simulink subsystem "Full_Generator"  (R2020a)
settings: Solver=VariableStepAuto  StartTime=0.0  StopTime=10.0  RelTol=1e-3
undefined symbols (not defined in the file): radps2rpm, torque_pu2Nm, WT_Params
libraries: powerlib x8, Generator_Lib x3, fl_lib x2, Full_Generator_Lib x1, nesl_utility x1
settings Model: Creator=Luke  LastModifiedBy=Luke

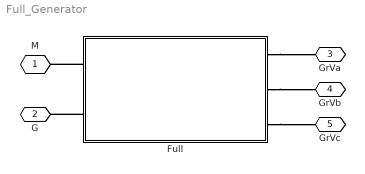
== system Full_Generator ==
  Full : Subsystem
  M : PMIOPort  Tag=PMCPort  Side=Left
  G : PMIOPort  Port=2  Side=Left
  GrVa : PMIOPort  Port=3  Side=Right
  GrVb : PMIOPort  Port=4  Side=Right
  GrVc : PMIOPort  Port=5  Side=Right
  connections:
  Full/RConn1 -- GrVa/RConn1
  Full/RConn2 -- GrVb/RConn1
  Full/RConn3 -- GrVc/RConn1
  Full/LConn1 -- M/RConn1
  Full/LConn2 -- G/RConn1

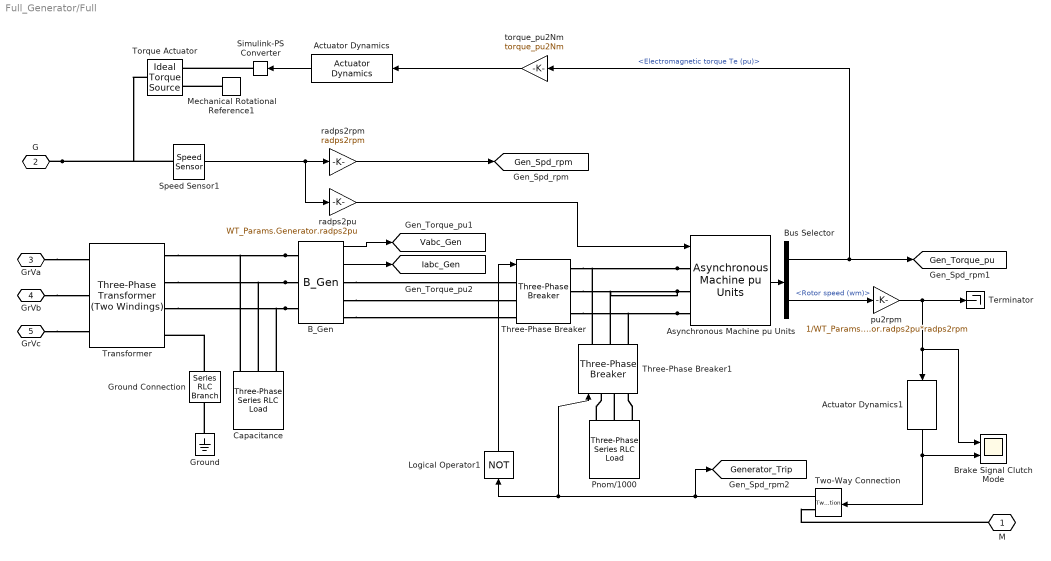
== system Full_Generator/Full ==
  Actuator Dynamics : Generator_Lib/Simple/Actuator Dynamics  b=WT_Params.Generator.generator_time_constant  x_initial=0
  Actuator Dynamics1 : Generator_Lib/Simple/Actuator Dynamics  b=WT_Params.Generator.generator_time_constant  x_initial=0
  Asynchronous Machine pu Units : powerlib/Machines/Asynchronous Machine pu Units  RotorType=Squirrel-cage  PresetModel=No  MechanicalLoad=Speed w  ShowDetailedParameters=on  ReferenceFrame=Rotor  Units=pu  MeasurementBus=off  NominalParameters=|  Stator=|  Rotor=|  Cage1=[0.01909 0.0397]  Cage2=[0.01909 0.0397]  Lm=WT_Params.Generator.mutual_inductance  Mechanical=[0.09526 0.05479 2]  PolePairs=2  InitialConditions=[1 0 0 0 0 0 0 0]  SimulateSaturation=off  Saturation="[0.212,0.4201,0.8125,1.0979,1.4799,2.2457,3.2586,4.5763,6.4763 ;   0.5,0.7,0.9,1,1.1,1.2 ,1.3,1.4,1.5]"  LoadFlowParameters=0  TsPowergui=0  TsBlock=-1  IterativeModel=Trapezoidal non iterative  IterativeDiscreteModel=Trapezoidal non iterative  Pmec=0
      NominalParameters=|
      | [WT_Params.Generator.nominal_power WT_Params.Generator.voltage
      | WT_Params.Generator.frequency]
      Stator=|
      | [WT_Params.Generator.Stator.resistance
      | WT_Params.Generator.Stator.inductance]
      Rotor=|
      | [WT_Params.Generator.Rotor.resistance
      | WT_Params.Generator.Rotor.inductance]
      settings: SourceProductBaseCode=PS
  B_Gen : Full_Generator_Lib/Full/B_Gen
      settings: SourceProductBaseCode=PS
  Brake Signal Clutch Mode : Scope  NumInputPorts=2
  Bus Selector : BusSelector  OutputSignals=Mechanical.Electromagnetic torque Te (pu),Mechanical.Rotor speed (wm)
  "Capacitance " : powerlib/Elements/Three-Phase Series RLC Load  LConnTagsString=A|B|C  Configuration=Delta  NominalVoltage=WT_Params.Generator.voltage  Vabc=[1e3 1e3 1e3]  Vabcp=[1e3 1e3 1e3]  NominalFrequency=WT_Params.Generator.frequency  UnbalancedPower=off  ActivePower=0  InductivePower=0  CapacitivePower=220e3  Pabc=[10e3 9e3 11e3]  QLabc=[100 90 110]  QCabc=[100 90 110]  Pabcp=[10e3 9e3 11e3]  QLabcp=[100 90 110]  QCabcp=[100 90 110]  Measurements=None  LoadType=constant Z
  Ground : powerlib/Elements/Ground  LConnTagsString=a
  Ground Connection : powerlib/Elements/Series RLC Branch  LConnTagsString=__new0  RConnTagsString=__new0  BranchType=R  Resistance=10  Inductance=1e-3  SetiL0=off  InitialCurrent=0  Capacitance=1e-6  Setx0=off  InitialVoltage=0  Measurements=None
  Logical Operator1 : Logic  Operator=NOT  AllPortsSameDT=off  OutDataTypeStr=float('double')
  Mechanical Rotational Reference1 : fl_lib/Mechanical/Rotational Elements/Mechanical Rotational Reference
  Pnom/1000 : powerlib/Elements/Three-Phase Series RLC Load  LConnTagsString=A|B|C  Configuration=Y (grounded)  NominalVoltage=WT_Params.Generator.voltage  Vabc=[1e3 1e3 1e3]  Vabcp=[1e3 1e3 1e3]  NominalFrequency=WT_Params.Generator.frequency  UnbalancedPower=off  ActivePower=WT_Params.Generator.nominal_power  InductivePower=0  CapacitivePower=0  Pabc=[10e3 9e3 11e3]  QLabc=[100 90 110]  QCabc=[100 90 110]  Pabcp=[10e3 9e3 11e3]  QLabcp=[100 90 110]  QCabcp=[100 90 110]  Measurements=None  LoadType=constant Z
  Simulink-PS Converter : nesl_utility/Simulink-PS Converter  PhysicalDomain=network_engine_domain  SubClassName=ps_input  LeftPortType=input  RightPortType=output  PseudoPeriodic=off  Frequencies=[]  NoiseDistribution=none  NoiseParameters=[]  Unit=1  AffineConversion=off  FilteringAndDerivatives=provide  SimscapeFilterOrder=1  InputFilterTimeConstant=0.001  UdotUserProvided=0
  Speed Sensor1 : Generator_Lib/Simple/Speed Sensor  SystemSampleTime=-1  Latency=0  AutoFrameSizeCalculation=off
  Terminator : Terminator
  Three-Phase Breaker : powerlib/Elements/Three-Phase Breaker  InitialState=closed  SwitchA=on  SwitchB=on  SwitchC=on  SwitchTimes="[1/60  5/60]"  External=on  BreakerResistance=WT_Params.Generator.Breakers.ron  SnubberResistance=WT_Params.Generator.Breakers.rp  SnubberCapacitance=WT_Params.Generator.Breakers.cp  Measurements=None
  Three-Phase Breaker1 : powerlib/Elements/Three-Phase Breaker  InitialState=open  SwitchA=on  SwitchB=on  SwitchC=on  SwitchTimes="[1/60  5/60]"  External=on  BreakerResistance=WT_Params.Generator.Breakers.ron  SnubberResistance=WT_Params.Generator.Breakers.rp  SnubberCapacitance=WT_Params.Generator.Breakers.cp  Measurements=None
  Torque Actuator : fl_lib/Mechanical/Mechanical Sources/Ideal Torque Source
  Transformer : powerlib/Elements/Three-Phase Transformer (Two Windings)  Winding1Connection=Yg  Winding2Connection=Yn  CoreType=Three single-phase transformers  SetSaturation=off  Hysteresis=off  DataFile='hysteresis'  SetInitialFlux=off  Measurements=None  UNITS=pu  NominalPower=[2e6 60]  Winding1=|  Winding2=[WT_Params.Generator.voltage, 0.025/30 , 0.025]  Rm=500  Lm=inf  L0=0.5  Saturation=[ 0,0 ; 0.0024,1.2 ; 1.0,1.52 ]  InitialFluxes=[ 0.8 , -0.8 , 0.7 ]  BreakLoop=off  DiscreteSolver=Trapezoidal iterative  DataType=off  TransfoNumber=1
      | [WT_Params.Grid.voltage, 0.025/30 ,
      | 0.025]
  Two-Way Connection : TwoWayConnection
  pu2rpm : Gain  Gain=1/WT_Params.Generator.radps2pu*radps2rpm
  radps2pu : Gain  Gain=WT_Params.Generator.radps2pu
  radps2rpm : Gain  Gain=radps2rpm
  torque_pu2Nm : Gain  Gain=torque_pu2Nm
  M : PMIOPort  Tag=PMCPort  Side=Left
  G : PMIOPort  Port=2  Side=Left
  GrVa : PMIOPort  Port=3  Side=Right
  GrVb : PMIOPort  Port=4  Side=Right
  GrVc : PMIOPort  Port=5  Side=Right
  tag scope: Gen_Spd_rpm=global, Gen_Torque_pu=global, Generator_Trip=global, Iabc_Gen=global, Vabc_Gen=global
  wires:
  Two-Way Connection/1 -> [Generator_Trip], Three-Phase Breaker1/1, Logical Operator1/1
  Speed Sensor1/1 -> radps2rpm/1, radps2pu/1
  torque_pu2Nm/1 -> Actuator Dynamics/1
  Bus Selector/2 -> pu2rpm/1  "<Rotor speed (wm)>"
  pu2rpm/1 -> Brake Signal Clutch Mode/1, Actuator Dynamics1/1, Terminator/1
  radps2rpm/1 -> [Gen_Spd_rpm]
  Logical Operator1/1 -> Three-Phase Breaker/1
  Actuator Dynamics/1 -> Simulink-PS Converter/1
  Asynchronous Machine pu Units/1 -> Bus Selector/1
  radps2pu/1 -> Asynchronous Machine pu Units/1
  B_Gen/2 -> [Iabc_Gen]
  Bus Selector/1 -> [Gen_Torque_pu], torque_pu2Nm/1  "<Electromagnetic torque Te (pu)>"
  B_Gen/1 -> [Vabc_Gen]
  Actuator Dynamics1/1 -> Two-Way Connection/1, Brake Signal Clutch Mode/2
  connections:
  Asynchronous Machine pu Units/LConn3 -- Three-Phase Breaker/RConn3 -- Three-Phase Breaker1/RConn3
  G/RConn1 -- Torque Actuator/LConn1 -- Speed Sensor1/LConn1
  Asynchronous Machine pu Units/LConn1 -- Three-Phase Breaker/RConn1 -- Three-Phase Breaker1/RConn1
  B_Gen/LConn3 -- Transformer/RConn3 -- "Capacitance "/LConn3
  B_Gen/LConn1 -- Transformer/RConn1 -- "Capacitance "/LConn1
  Asynchronous Machine pu Units/LConn2 -- Three-Phase Breaker/RConn2 -- Three-Phase Breaker1/RConn2
  B_Gen/LConn2 -- Transformer/RConn2 -- "Capacitance "/LConn2
  M/RConn1 -- Two-Way Connection/RConn1
  GrVc/RConn1 -- Transformer/LConn3
  B_Gen/RConn2 -- Three-Phase Breaker/LConn2
  Ground/LConn1 -- Ground Connection/RConn1
  B_Gen/RConn3 -- Three-Phase Breaker/LConn3
  Mechanical Rotational Reference1/LConn1 -- Torque Actuator/RConn2
  B_Gen/RConn1 -- Three-Phase Breaker/LConn1
  Pnom/1000/LConn3 -- Three-Phase Breaker1/LConn3
  Pnom/1000/LConn2 -- Three-Phase Breaker1/LConn2
  Pnom/1000/LConn1 -- Three-Phase Breaker1/LConn1
  Ground Connection/LConn1 -- Transformer/RConn4
  Simulink-PS Converter/RConn1 -- Torque Actuator/RConn1
  GrVb/RConn1 -- Transformer/LConn2
  GrVa/RConn1 -- Transformer/LConn1
